simulink model "Battery_droop_control_2"  (R2022a)
settings: Solver=ode23tb  StartTime=0.0  StopTime=1  RelTol=1e-3  EnableMultiTasking=on
values from neighbouring files (symbols this model uses):
  R_power_mode_load_change = zeros(1, length(load_percent_list))    [Battery_charge_discharge_FSBB_param_init.m]
  R_voltage_mode_load_change = zeros(1, length(load_percent_list))    [Battery_charge_discharge_FSBB_param_init.m]
  time_step = 1 / wave_freq    (= 2.22222222222e-05)    [Battery_charge_discharge_FSBB_param_init.m]
undefined symbols (not defined in the file or in its folder): Ion, Lithium
libraries: spsSeriesRLCBranchLib x26, spsTriangleGeneratorLib x16, slpidlib x13, spsCurrentMeasurementLib x9, spsIGBTDiodeLib x8, spsIdealSwitchLib x8, spsVoltageMeasurementLib x8, simulink x4, spsBatteryLib x3, spsControlledVoltageSourceLib x3, spspowerguiLib x1, spsDCVoltageSourceLib x1
(part 1 of 4)
settings Model: Creator=Lei  LastModifiedBy=zhang
settings SolverCC: AlgebraicLoopSolver=TrustRegion
settings DataIOCC: LimitDataPoints=on  SaveFormat=Array  ReturnWorkspaceOutputs=off
settings OptimizationCC: LifeSpan=inf
settings DebuggingCC: SolverPrmCheckMsg=warning  UnconnectedInputMsg=warning  UnconnectedOutputMsg=warning  UnconnectedLineMsg=warning  SFUnexpectedBacktrackingDiag=warning  SFNoUnconditionalDefaultTransitionDiag=warning  SFExecutionAtInitializationDiag=none  SFMachineParentedDataDiag=warning  ArithmeticOperatorsInVariantConditions=warning
settings HardwareCC: ProdBitPerPointer=32  ProdBitPerSizeT=32  ProdBitPerPtrDiffT=32  ProdLargestAtomicFloat=None  ProdIntDivRoundTo=Undefined  ProdEndianess=Unspecified  ProdWordSize=32  ProdHWDeviceType=32-bit Generic
settings ModelReferenceCC: PropagateSignalLabelsOutOfModel=off
settings SFSimCC: SimUseLocalCustomCode=off  CustomCodeUndefinedFunction=UseInterfaceOnly
settings RTWCC: RTWUseLocalCustomCode=off
settings CodeAppCC: StateflowObjectComments=on
settings GRTTargetCC: TargetLangStandard=C89/C90 (ANSI)
settings ConfigComp: CovMetricSettings=dw  CovSaveCumulativeToWorkspaceVar=on  CovSaveSingleToWorkspaceVar=on  CovExternalEMLEnable=off  CovSFcnEnable=off
settings SimscapeCC: SimscapeNormalizeSystem=off

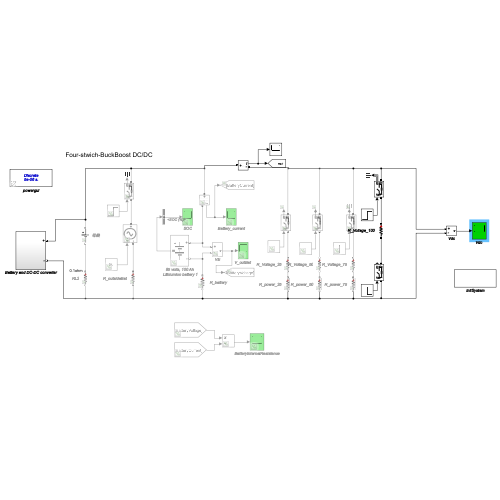
[thumbnail: Simulink's stored preview of the top-level diagram]
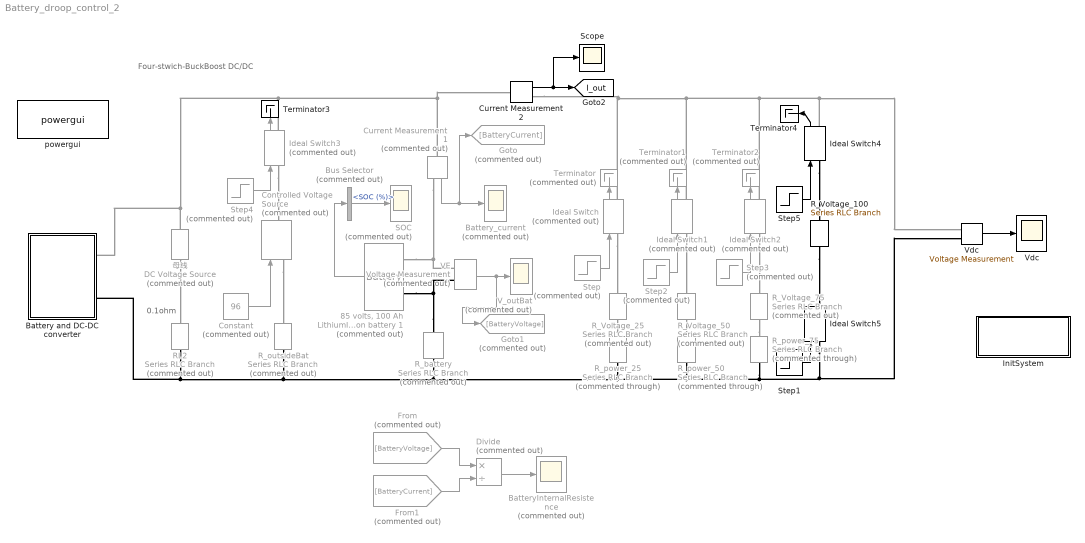
== system Battery_droop_control_2 ==
  note: 0.1ohm
  note: Four-stwich-BuckBoost DC/DC
  "85 volts, 100 Ah LithiumIon battery 1" : spsBatteryLib/Battery  Commented=on  BatType=Lithium-Ion  ShowTempParam=off  ThermalPreset=no  ShowAgeParam=off  NomV=85  NomQ=100  SOC=10  Batt_Tr=30  PresetModel=off  MaxQ=107.6923  MinV=83.2  FullV=115.2  Dis_rate=43.4783  R=0.08  Normal_OP=96.1538  expZone=[92.2034, 20]  current=[6.5 13 32.5]  Units=Time  Tci=20  NomT=20  T2=-30  MaxQ2=4.8  FullV2=7.1  Normal_OP2=5.655  expZone2="[6.58           1]"  Rca=0.6  ti=2000  Dp=0  Neq0=0  Tsim=1e6  Ta1=25  Qeol=5.4*0.9  Reol=0.013333*1.2  Char_age=[2.3478, 3]  Dis_age=[2.3478, 10]  N1=1500  N2=10500  N3=1000  N4=1400  Ta2=45  N5=950
  Battery and DC-DC converter : Subsystem
  BatteryInternalResistence : Scope  Commented=on
  Battery_current : Scope  Commented=on
  Bus Selector : BusSelector  Commented=on  OutputSignals=SOC (%)
  Constant : Constant  Commented=on  Value=96
  Controlled Voltage Source : spsControlledVoltageSourceLib/Controlled Voltage Source  Commented=on  Initialize=on  Source_Type=DC  Amplitude=96  Phase=0  Frequency=0  Measurements=None
  Current Measurement1 : spsCurrentMeasurementLib/Current Measurement  Commented=on  PhasorSimulation=off  OutputType=Complex  PSBequivalent=0
  Current Measurement2 : spsCurrentMeasurementLib/Current Measurement  PhasorSimulation=off  OutputType=Complex  PSBequivalent=0
  Divide : Product  Commented=on  Inputs=*/
  From : From  Commented=on  GotoTag=BatteryVoltage
  From1 : From  Commented=on  GotoTag=BatteryCurrent
  Goto : Goto  Commented=on  GotoTag=BatteryCurrent
  Goto1 : Goto  Commented=on  GotoTag=BatteryVoltage
  Ideal Switch{,1..3} (4 alike) : spsIdealSwitchLib/Ideal Switch  Commented=on  Ron=0.001  Lon=0  IC=0  Rs=1e5  Cs=inf  Measurements=on
  Ideal Switch4 : spsIdealSwitchLib/Ideal Switch  Ron=0.001  Lon=0  IC=0  Rs=1e5  Cs=inf  Measurements=on
  Ideal Switch5 : spsIdealSwitchLib/Ideal Switch  Ron=0.001  Lon=0  IC=0  Rs=1e5  Cs=inf  Measurements=on
  InitSystem : Subsystem
      settings: OpenFcn=Battery_charge_discharge_FSBB_param_init
  RL2 : spsSeriesRLCBranchLib/Series RLC Branch  Commented=on  LConnTagsString=__new0  RConnTagsString=__new0  BranchType=R  Resistance=0.1  Inductance=1e-3  SetiL0=off  InitialCurrent=0  Capacitance=1e-6  Setx0=off  InitialVoltage=0  Measurements=None
  R_Voltage_100 : spsSeriesRLCBranchLib/Series RLC Branch  LConnTagsString=__new0  RConnTagsString=__new0  BranchType=R  Resistance=R_voltage_mode_load_change(4)  Inductance=1e-3  SetiL0=off  InitialCurrent=0  Capacitance=1e-6  Setx0=off  InitialVoltage=0  Measurements=None
  R_Voltage_25 : spsSeriesRLCBranchLib/Series RLC Branch  Commented=on  LConnTagsString=__new0  RConnTagsString=__new0  BranchType=R  Resistance=R_voltage_mode_load_change(1)* 10  Inductance=1e-3  SetiL0=off  InitialCurrent=0  Capacitance=1e-6  Setx0=off  InitialVoltage=0  Measurements=None
  R_Voltage_50 : spsSeriesRLCBranchLib/Series RLC Branch  Commented=on  LConnTagsString=__new0  RConnTagsString=__new0  BranchType=R  Resistance=R_voltage_mode_load_change(2)  Inductance=1e-3  SetiL0=off  InitialCurrent=0  Capacitance=1e-6  Setx0=off  InitialVoltage=0  Measurements=None
  R_Voltage_75 : spsSeriesRLCBranchLib/Series RLC Branch  Commented=on  LConnTagsString=__new0  RConnTagsString=__new0  BranchType=R  Resistance=R_voltage_mode_load_change(3)  Inductance=1e-3  SetiL0=off  InitialCurrent=0  Capacitance=1e-6  Setx0=off  InitialVoltage=0  Measurements=None
  R_battery : spsSeriesRLCBranchLib/Series RLC Branch  Commented=on  LConnTagsString=__new0  RConnTagsString=__new0  BranchType=R  Resistance=0.1  Inductance=1e-3  SetiL0=off  InitialCurrent=0  Capacitance=1440e-6  Setx0=off  InitialVoltage=80  Measurements=None
  R_outsideBat : spsSeriesRLCBranchLib/Series RLC Branch  Commented=on  LConnTagsString=__new0  RConnTagsString=__new0  BranchType=R  Resistance=0.1  Inductance=1e-3  SetiL0=off  InitialCurrent=0  Capacitance=1e-6  Setx0=off  InitialVoltage=0  Measurements=None
  R_power_25 : spsSeriesRLCBranchLib/Series RLC Branch  Commented=through  LConnTagsString=__new0  RConnTagsString=__new0  BranchType=R  Resistance=R_power_mode_load_change(1)  Inductance=1e-3  SetiL0=off  InitialCurrent=0  Capacitance=1e-6  Setx0=off  InitialVoltage=0  Measurements=None
  R_power_50 : spsSeriesRLCBranchLib/Series RLC Branch  Commented=through  LConnTagsString=__new0  RConnTagsString=__new0  BranchType=R  Resistance=R_power_mode_load_change(2)  Inductance=1e-3  SetiL0=off  InitialCurrent=0  Capacitance=1e-6  Setx0=off  InitialVoltage=0  Measurements=None
  R_power_75 : spsSeriesRLCBranchLib/Series RLC Branch  Commented=through  LConnTagsString=__new0  RConnTagsString=__new0  BranchType=R  Resistance=R_power_mode_load_change(3)  Inductance=1e-3  SetiL0=off  InitialCurrent=0  Capacitance=1e-6  Setx0=off  InitialVoltage=0  Measurements=None
  SOC : Scope  Commented=on
  Scope : Scope
  Step : Step  Commented=on  Time=0.3  SampleTime=0
  Step1 : Step  Time=0.5  Before=1  After=0  SampleTime=0
  Step2 : Step  Commented=on  Time=0.3  SampleTime=0
  Step3 : Step  Commented=on  Time=0.3  SampleTime=0
  Step4 : Step  Commented=on  Time=0.3  Before=1  SampleTime=0
  Step5 : Step  Time=0  SampleTime=0
  Terminator : Terminator  Commented=on
  Terminator1 : Terminator  Commented=on
  Terminator2 : Terminator  Commented=on
  Terminator3 : Terminator
  Terminator4 : Terminator
  VE : spsVoltageMeasurementLib/Voltage Measurement  Commented=on  PhasorSimulation=off  OutputType=Complex  PSBequivalent=0
  "V_outBat " : Scope  Commented=on
  Vdc : spsVoltageMeasurementLib/Voltage Measurement  PhasorSimulation=off  OutputType=Complex  PSBequivalent=0
  "Vdc " : Scope
  powergui : spspowerguiLib/powergui  Priority=1  SimulationMode=Discrete  SampleTime=5e-6  frequency=60  Iterations=50  frequencyindice=0  Pbase=100e6  ErrMax=1e-4  UnitsV=kV  UnitsW=MW  buscounter=0  FunctionMessages=off  echomessages=off  EnableUseOfTLC=off  CurrentSourceSwitches=off  DisableSnubberDevices=off  DisableRonSwitches=off  DisableVfSwitches=off  DisplayEquations=off  AutomaticDiscreteSolvers=off  SolverType=Tustin/Backward Euler (TBE)  Interpol=off  ExternalGateDelay=off  methode=off  Ts=100  x0status=blocks  SPID=off  SwTol=0  HookPort=off  NonlinearTolerance=1e-4  nMaxIteration=100  ContinueOnMaxIteration=off  RestoreLinks=warning  ResistiveCurrentMeasurement=off  Frange=[0:2:500]  Ylog=off  Xlog=on  ShowGrid=off  save=off  variable=ZData  structure=0  ZoomFFT=off  StartTime=0.0  cycles=1  DisplayStyle=1  fundamental=60  FreqAxis=off  MaxFrequency=1000  frequencyindicesteady=1  RmsSteady=1  display=off
  "母线  " : spsDCVoltageSourceLib/DC Voltage Source  Commented=on  Amplitude=109  Measurements=None
  tag scope: I_out=global
  wires:
  Vdc/1 -> "Vdc "/1
  From/1 -> Divide/1
  From1/1 -> Divide/2
  Divide/1 -> BatteryInternalResistence/1
  Current Measurement1/1 -> Goto/1, Battery_current/1
  Step1/1 -> Ideal Switch5/1
  Ideal Switch1/1 -> Terminator1/1
  Step4/1 -> Ideal Switch3/1
  Step5/1 -> Ideal Switch4/1
  Ideal Switch3/1 -> Terminator3/1
  Current Measurement2/1 -> [I_out], Scope/1
  Step/1 -> Ideal Switch/1
  Ideal Switch/1 -> Terminator/1
  Ideal Switch2/1 -> Terminator2/1
  VE/1 -> "V_outBat "/1, Goto1/1
  Step3/1 -> Ideal Switch2/1
  Ideal Switch4/1 -> Terminator4/1
  Step2/1 -> Ideal Switch1/1
  "85 volts, 100 Ah LithiumIon battery 1"/1 -> Bus Selector/1
  Bus Selector/1 -> SOC/1  "<SOC (%)>"
  Constant/1 -> Controlled Voltage Source/1
  connections:
  "85 volts, 100 Ah LithiumIon battery 1"/LConn1 -- VE/LConn1 -- Current Measurement1/RConn1
  Ideal Switch2/RConn1 -- Vdc/LConn1 -- Ideal Switch4/RConn1 -- Current Measurement2/RConn1 -- Ideal Switch/RConn1 -- Ideal Switch1/RConn1
  R_power_75/RConn1 -- Vdc/LConn2 -- Ideal Switch5/LConn1 -- R_power_50/RConn1 -- R_power_25/RConn1 -- R_battery/RConn1 -- Battery and DC-DC converter/RConn2 -- RL2/RConn1 -- R_outsideBat/RConn1
  "母线  "/RConn1 -- Battery and DC-DC converter/RConn1 -- Ideal Switch3/RConn1 -- Current Measurement1/LConn1 -- Current Measurement2/LConn1
  R_battery/LConn1 -- VE/LConn2 -- "85 volts, 100 Ah LithiumIon battery 1"/LConn2
  "母线  "/LConn1 -- RL2/LConn1
  R_Voltage_100/RConn1 -- Ideal Switch5/RConn1
  Ideal Switch/LConn1 -- R_Voltage_25/LConn1
  Ideal Switch1/LConn1 -- R_Voltage_50/LConn1
  Ideal Switch4/LConn1 -- R_Voltage_100/LConn1
  Controlled Voltage Source/LConn1 -- R_outsideBat/LConn1
  R_Voltage_25/RConn1 -- R_power_25/LConn1
  R_Voltage_50/RConn1 -- R_power_50/LConn1
  R_Voltage_75/RConn1 -- R_power_75/LConn1
  Ideal Switch2/LConn1 -- R_Voltage_75/LConn1
  Ideal Switch3/LConn1 -- Controlled Voltage Source/RConn1
